simulink model "Vehicle_Dyanamic_Model"  (R2020a)
settings: Solver=VariableStepAuto  StartTime=0.0  StopTime=10.0  RelTol=1e-3
undefined symbols (not defined in the file): h, km, m, s
libraries: aerolibconvert2 x2, simulink_extras x1
settings Model: Creator=akash  LastModifiedBy=akash

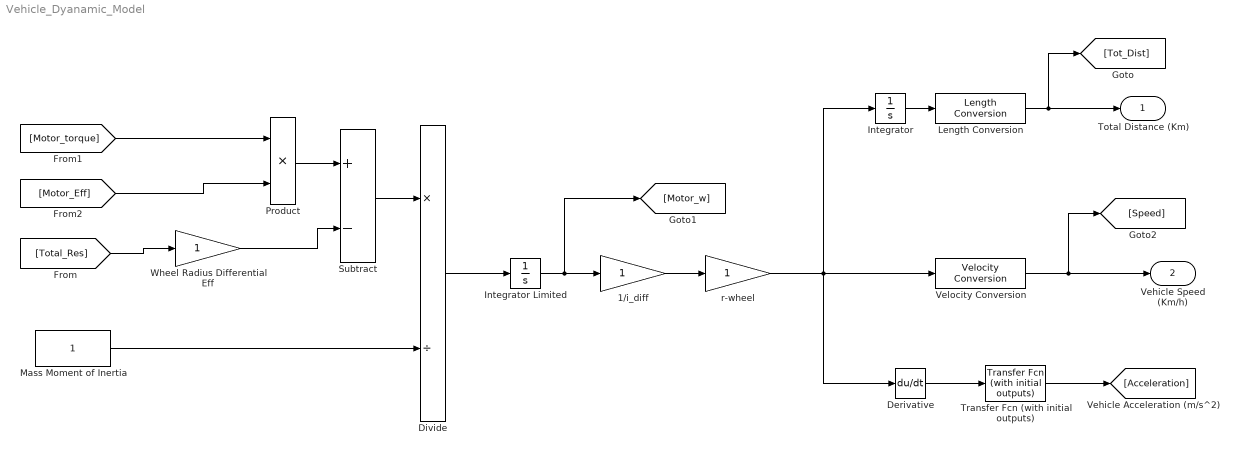
== system Vehicle_Dyanamic_Model ==
  1/i_diff : Gain
  Derivative : Derivative
  Divide : Product  Inputs=*/
  Integrator : Integrator
  Integrator Limited : Integrator  LimitOutput=on  UpperSaturationLimit=1  LowerSaturationLimit=0
  Length Conversion : aerolibconvert2/Length Conversion  IU=m  OU=km
  Mass Moment of Inertia : Constant
  Product : Product
  Subtract : Sum  Inputs=+-
  Transfer Fcn (with initial outputs) : simulink_extras/Additional Linear/Transfer Fcn (with initial outputs)  N=[1]  D="[0.01  1]"  Y0=.5  U0=0
  Velocity Conversion : aerolibconvert2/Velocity Conversion  IU=m/s  OU=km/h
  Wheel Radius Differential Eff : Gain
  r-wheel : Gain
  Total Distance (Km) : Outport
  "Vehicle Speed (Km/h) " : Outport  Port=2
  wires:
  [Motor_torque] -> Product/1
  [Motor_Eff] -> Product/2
  Product/1 -> Subtract/1
  Wheel Radius Differential Eff/1 -> Subtract/2
  [Total_Res] -> Wheel Radius Differential Eff/1
  Subtract/1 -> Divide/1
  Mass Moment of Inertia/1 -> Divide/2
  Divide/1 -> Integrator Limited/1
  Integrator Limited/1 -> 1/i_diff/1, [Motor_w]
  1/i_diff/1 -> r-wheel/1
  r-wheel/1 -> Velocity Conversion/1, Integrator/1, Derivative/1
  Integrator/1 -> Length Conversion/1
  Length Conversion/1 -> Total Distance (Km)/1, [Tot_Dist]
  Velocity Conversion/1 -> [Speed], "Vehicle Speed (Km/h) "/1
  Derivative/1 -> Transfer Fcn (with initial outputs)/1
  Transfer Fcn (with initial outputs)/1 -> [Acceleration]
